simulink model "extra2 - Copy"  (R2017a)
settings: Solver=VariableStepAuto  StartTime=0.0  StopTime=10.0  RelTol=1e-3
libraries: hdlsllib x20, simulink x10
settings Model: Creator=wachala.j  LastModifiedBy=wachala.j
settings OptimizationCC: BlockReduction=off  ConditionallyExecuteInputs=off  DefaultParameterBehavior=Inlined
settings DebuggingCC: AlgebraicLoopMsg=error
settings HardwareCC: ProdBitPerPointer=32  ProdBitPerSizeT=32  ProdBitPerPtrDiffT=32  ProdLargestAtomicFloat=None  ProdIntDivRoundTo=Undefined  ProdEndianess=Unspecified  ProdWordSize=32  ProdHWDeviceType=ASIC/FPGA->ASIC/FPGA  ProdEqTarget=off

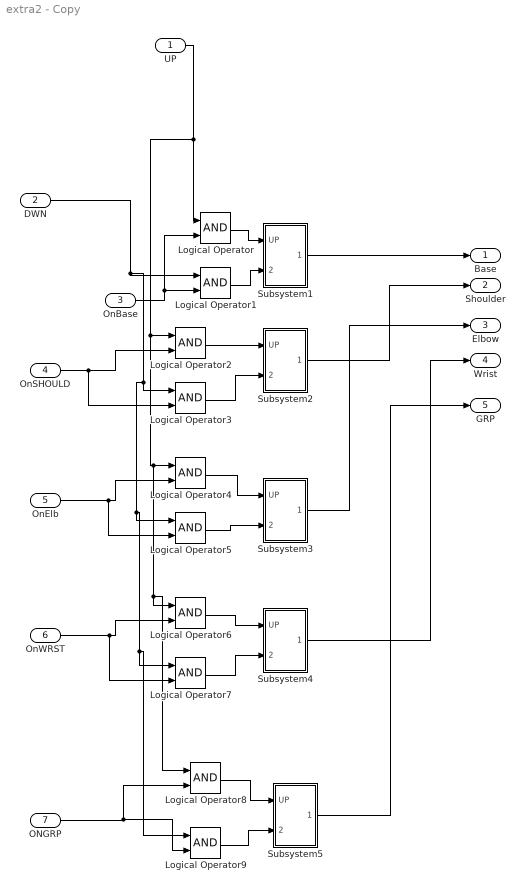
== system extra2 - Copy ==
  UP : Inport
  DWN : Inport  Port=2
  OnBase : Inport  Port=3
  OnSHOULD : Inport  Port=4
  OnElb : Inport  Port=5
  OnWRST : Inport  Port=6
  ONGRP : Inport  Port=7
  Logical Operator{,1..9} (10 alike) : Logic  AllPortsSameDT=off  OutDataTypeStr=boolean
  Subsystem1 : Subsystem
  Subsystem2 : Subsystem
  Subsystem3 : Subsystem
  Subsystem4 : Subsystem
  Subsystem5 : Subsystem
  Base : Outport  OutDataTypeStr=boolean
  "Shoulder " : Outport  Port=2  OutDataTypeStr=boolean
  Elbow : Outport  Port=3  OutDataTypeStr=boolean
  Wrist : Outport  Port=4  OutDataTypeStr=boolean
  GRP : Outport  Port=5  OutDataTypeStr=boolean
  wires:
  UP/1 -> Logical Operator8/1, Logical Operator6/1, Logical Operator4/1, Logical Operator2/1, Logical Operator/1
  OnBase/1 -> Logical Operator1/2, Logical Operator/2
  DWN/1 -> Logical Operator9/1, Logical Operator7/1, Logical Operator5/1, Logical Operator3/1, Logical Operator1/1
  Logical Operator1/1 -> Subsystem1/2(DWN)
  Logical Operator/1 -> Subsystem1/1(UP)
  Subsystem1/1(PWM) -> Base/1
  ONGRP/1 -> Logical Operator9/2, Logical Operator8/2
  OnWRST/1 -> Logical Operator7/2, Logical Operator6/2
  OnElb/1 -> Logical Operator5/2, Logical Operator4/2
  OnSHOULD/1 -> Logical Operator3/2, Logical Operator2/2
  Logical Operator8/1 -> Subsystem5/1(UP)
  Logical Operator9/1 -> Subsystem5/2(DWN)
  Logical Operator7/1 -> Subsystem4/2(DWN)
  Logical Operator6/1 -> Subsystem4/1(UP)
  Logical Operator5/1 -> Subsystem3/2(DWN)
  Logical Operator4/1 -> Subsystem3/1(UP)
  Logical Operator3/1 -> Subsystem2/2(DWN)
  Logical Operator2/1 -> Subsystem2/1(UP)
  Subsystem2/1(PWM) -> "Shoulder "/1
  Subsystem3/1(PWM) -> Elbow/1
  Subsystem4/1(PWM) -> Wrist/1
  Subsystem5/1(PWM) -> GRP/1

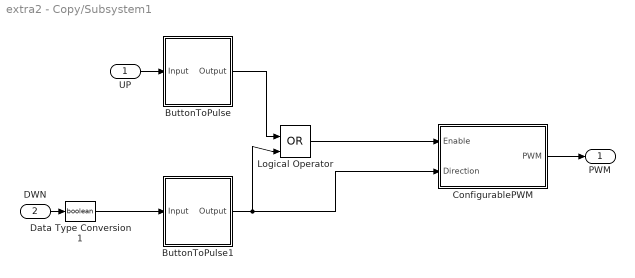
== system extra2 - Copy/Subsystem1 ==
  UP : Inport
  DWN : Inport  Port=2
  ButtonToPulse : Subsystem
  ButtonToPulse1 : Subsystem
  ConfigurablePWM : Subsystem
  Data Type Conversion1 : DataTypeConversion  OutDataTypeStr=boolean
  Logical Operator : Logic  Operator=OR  IconShape=distinctive  AllPortsSameDT=off  OutDataTypeStr=boolean
  PWM : Outport  OutDataTypeStr=boolean
  wires:
  ButtonToPulse1/1(Output) -> Logical Operator/2, ConfigurablePWM/2(Direction)
  Data Type Conversion1/1 -> ButtonToPulse1/1(Input)
  ButtonToPulse/1(Output) -> Logical Operator/1
  UP/1 -> ButtonToPulse/1(Input)
  DWN/1 -> Data Type Conversion1/1
  Logical Operator/1 -> ConfigurablePWM/1(Enable)
  ConfigurablePWM/1(PWM) -> PWM/1

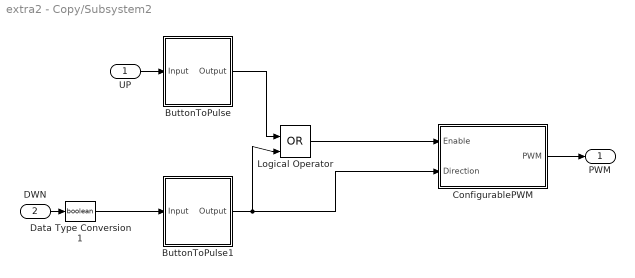
== system extra2 - Copy/Subsystem2 ==
  UP : Inport
  DWN : Inport  Port=2
  ButtonToPulse : Subsystem
  ButtonToPulse1 : Subsystem
  ConfigurablePWM : Subsystem
  Data Type Conversion1 : DataTypeConversion  OutDataTypeStr=boolean
  Logical Operator : Logic  Operator=OR  IconShape=distinctive  AllPortsSameDT=off  OutDataTypeStr=boolean
  PWM : Outport  OutDataTypeStr=boolean
  wires:
  ButtonToPulse1/1(Output) -> Logical Operator/2, ConfigurablePWM/2(Direction)
  Data Type Conversion1/1 -> ButtonToPulse1/1(Input)
  ButtonToPulse/1(Output) -> Logical Operator/1
  UP/1 -> ButtonToPulse/1(Input)
  DWN/1 -> Data Type Conversion1/1
  Logical Operator/1 -> ConfigurablePWM/1(Enable)
  ConfigurablePWM/1(PWM) -> PWM/1

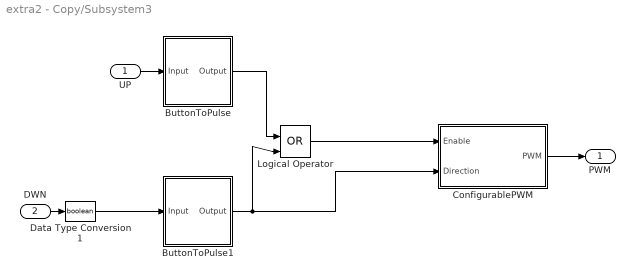
== system extra2 - Copy/Subsystem3 ==
  UP : Inport
  DWN : Inport  Port=2
  ButtonToPulse : Subsystem
  ButtonToPulse1 : Subsystem
  ConfigurablePWM : Subsystem
  Data Type Conversion1 : DataTypeConversion  OutDataTypeStr=boolean
  Logical Operator : Logic  Operator=OR  IconShape=distinctive  AllPortsSameDT=off  OutDataTypeStr=boolean
  PWM : Outport  OutDataTypeStr=boolean
  wires:
  ButtonToPulse1/1(Output) -> Logical Operator/2, ConfigurablePWM/2(Direction)
  Data Type Conversion1/1 -> ButtonToPulse1/1(Input)
  ButtonToPulse/1(Output) -> Logical Operator/1
  UP/1 -> ButtonToPulse/1(Input)
  DWN/1 -> Data Type Conversion1/1
  Logical Operator/1 -> ConfigurablePWM/1(Enable)
  ConfigurablePWM/1(PWM) -> PWM/1

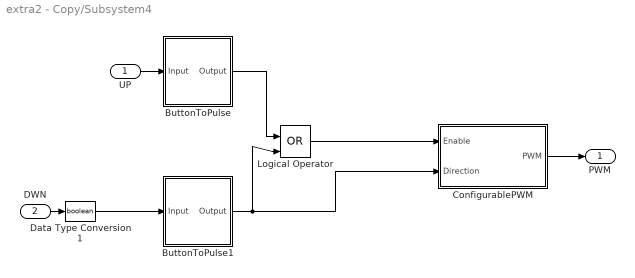
== system extra2 - Copy/Subsystem4 ==
  UP : Inport
  DWN : Inport  Port=2
  ButtonToPulse : Subsystem
  ButtonToPulse1 : Subsystem
  ConfigurablePWM : Subsystem
  Data Type Conversion1 : DataTypeConversion  OutDataTypeStr=boolean
  Logical Operator : Logic  Operator=OR  IconShape=distinctive  AllPortsSameDT=off  OutDataTypeStr=boolean
  PWM : Outport  OutDataTypeStr=boolean
  wires:
  ButtonToPulse1/1(Output) -> Logical Operator/2, ConfigurablePWM/2(Direction)
  Data Type Conversion1/1 -> ButtonToPulse1/1(Input)
  ButtonToPulse/1(Output) -> Logical Operator/1
  UP/1 -> ButtonToPulse/1(Input)
  DWN/1 -> Data Type Conversion1/1
  Logical Operator/1 -> ConfigurablePWM/1(Enable)
  ConfigurablePWM/1(PWM) -> PWM/1

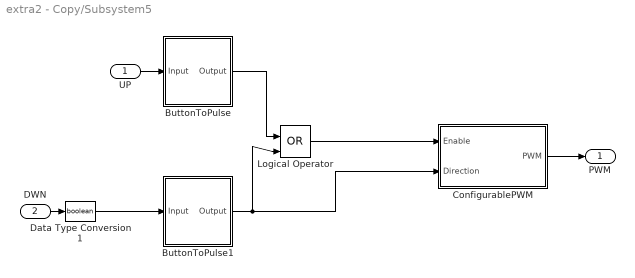
== system extra2 - Copy/Subsystem5 ==
  UP : Inport
  DWN : Inport  Port=2
  ButtonToPulse : Subsystem
  ButtonToPulse1 : Subsystem
  ConfigurablePWM : Subsystem
  Data Type Conversion1 : DataTypeConversion  OutDataTypeStr=boolean
  Logical Operator : Logic  Operator=OR  IconShape=distinctive  AllPortsSameDT=off  OutDataTypeStr=boolean
  PWM : Outport  OutDataTypeStr=boolean
  wires:
  ButtonToPulse1/1(Output) -> Logical Operator/2, ConfigurablePWM/2(Direction)
  Data Type Conversion1/1 -> ButtonToPulse1/1(Input)
  ButtonToPulse/1(Output) -> Logical Operator/1
  UP/1 -> ButtonToPulse/1(Input)
  DWN/1 -> Data Type Conversion1/1
  Logical Operator/1 -> ConfigurablePWM/1(Enable)
  ConfigurablePWM/1(PWM) -> PWM/1

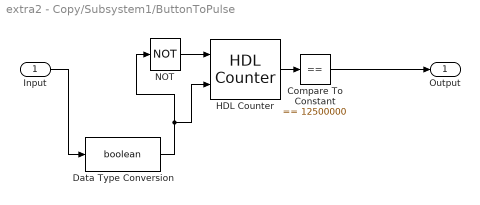
== system extra2 - Copy/Subsystem1/ButtonToPulse ==
  Input : Inport
  Compare To Constant : simulink/Logic and Bit Operations/Compare To Constant  relop===  const=12500000  OutDataTypeStr=boolean
  Data Type Conversion : DataTypeConversion  OutDataTypeStr=boolean
  HDL Counter : hdlsllib/HDL Operations/HDL Counter  CountType=Count limited  CountInit=0  CountStep=1  CountMax=50000000  CountFromType=Initial value  CountFrom=0  CountResetPort=on  CountLoadPort=off  CountEnbPort=on  CountDirPort=off  CountDataType=Unsigned  CountWordLen=32  CountFracLen=0  CountSampTime=1
      settings: SourceProductName=HDL Coder  SourceProductBaseCode=HD
  NOT : Logic  Operator=NOT  IconShape=distinctive  AllPortsSameDT=off  OutDataTypeStr=boolean
  Output : Outport
  wires:
  NOT/1 -> HDL Counter/1
  Data Type Conversion/1 -> HDL Counter/2, NOT/1
  HDL Counter/1 -> Compare To Constant/1
  Input/1 -> Data Type Conversion/1
  Compare To Constant/1 -> Output/1

== system extra2 - Copy/Subsystem1/ButtonToPulse1 ==
  Input : Inport
  Compare To Constant : simulink/Logic and Bit Operations/Compare To Constant  relop===  const=12500000  OutDataTypeStr=boolean
  Data Type Conversion : DataTypeConversion  OutDataTypeStr=boolean
  HDL Counter : hdlsllib/HDL Operations/HDL Counter  CountType=Count limited  CountInit=0  CountStep=1  CountMax=50000000  CountFromType=Initial value  CountFrom=0  CountResetPort=on  CountLoadPort=off  CountEnbPort=on  CountDirPort=off  CountDataType=Unsigned  CountWordLen=32  CountFracLen=0  CountSampTime=1
      settings: SourceProductName=HDL Coder  SourceProductBaseCode=HD
  NOT : Logic  Operator=NOT  IconShape=distinctive  AllPortsSameDT=off  OutDataTypeStr=boolean
  Output : Outport
  wires:
  NOT/1 -> HDL Counter/1
  Data Type Conversion/1 -> HDL Counter/2, NOT/1
  HDL Counter/1 -> Compare To Constant/1
  Input/1 -> Data Type Conversion/1
  Compare To Constant/1 -> Output/1

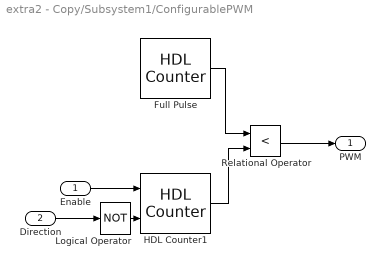
== system extra2 - Copy/Subsystem1/ConfigurablePWM ==
  Enable : Inport  OutDataTypeStr=boolean
  Direction : Inport  Port=2  OutDataTypeStr=boolean
  Full Pulse : hdlsllib/HDL Operations/HDL Counter  CountType=Count limited  CountInit=0  CountStep=1  CountMax=1000000  CountFromType=Initial value  CountFrom=0  CountResetPort=off  CountLoadPort=off  CountEnbPort=off  CountDirPort=off  CountDataType=Unsigned  CountWordLen=32  CountFracLen=0  CountSampTime=1
      settings: SourceProductName=HDL Coder  SourceProductBaseCode=HD
  HDL Counter1 : hdlsllib/HDL Operations/HDL Counter  CountType=Count limited  CountInit=30000  CountStep=6000  CountMax=120000  CountFromType=Initial value  CountFrom=30000  CountResetPort=off  CountLoadPort=off  CountEnbPort=on  CountDirPort=on  CountDataType=Unsigned  CountWordLen=32  CountFracLen=0  CountSampTime=1
      settings: SourceProductName=HDL Coder  SourceProductBaseCode=HD
  Logical Operator : Logic  Operator=NOT  IconShape=distinctive  AllPortsSameDT=off  OutDataTypeStr=boolean
  Relational Operator : RelationalOperator  Operator=<  OutDataTypeStr=boolean  RndMeth=Simplest
  PWM : Outport
  wires:
  Relational Operator/1 -> PWM/1
  HDL Counter1/1 -> Relational Operator/2
  Full Pulse/1 -> Relational Operator/1
  Enable/1 -> HDL Counter1/1
  Direction/1 -> Logical Operator/1
  Logical Operator/1 -> HDL Counter1/2

== system extra2 - Copy/Subsystem2/ButtonToPulse ==
  Input : Inport
  Compare To Constant : simulink/Logic and Bit Operations/Compare To Constant  relop===  const=12500000  OutDataTypeStr=boolean
  Data Type Conversion : DataTypeConversion  OutDataTypeStr=boolean
  HDL Counter : hdlsllib/HDL Operations/HDL Counter  CountType=Count limited  CountInit=0  CountStep=1  CountMax=50000000  CountFromType=Initial value  CountFrom=0  CountResetPort=on  CountLoadPort=off  CountEnbPort=on  CountDirPort=off  CountDataType=Unsigned  CountWordLen=32  CountFracLen=0  CountSampTime=1
      settings: SourceProductName=HDL Coder  SourceProductBaseCode=HD
  NOT : Logic  Operator=NOT  IconShape=distinctive  AllPortsSameDT=off  OutDataTypeStr=boolean
  Output : Outport
  wires:
  NOT/1 -> HDL Counter/1
  Data Type Conversion/1 -> HDL Counter/2, NOT/1
  HDL Counter/1 -> Compare To Constant/1
  Input/1 -> Data Type Conversion/1
  Compare To Constant/1 -> Output/1

== system extra2 - Copy/Subsystem2/ButtonToPulse1 ==
  Input : Inport
  Compare To Constant : simulink/Logic and Bit Operations/Compare To Constant  relop===  const=12500000  OutDataTypeStr=boolean
  Data Type Conversion : DataTypeConversion  OutDataTypeStr=boolean
  HDL Counter : hdlsllib/HDL Operations/HDL Counter  CountType=Count limited  CountInit=0  CountStep=1  CountMax=50000000  CountFromType=Initial value  CountFrom=0  CountResetPort=on  CountLoadPort=off  CountEnbPort=on  CountDirPort=off  CountDataType=Unsigned  CountWordLen=32  CountFracLen=0  CountSampTime=1
      settings: SourceProductName=HDL Coder  SourceProductBaseCode=HD
  NOT : Logic  Operator=NOT  IconShape=distinctive  AllPortsSameDT=off  OutDataTypeStr=boolean
  Output : Outport
  wires:
  NOT/1 -> HDL Counter/1
  Data Type Conversion/1 -> HDL Counter/2, NOT/1
  HDL Counter/1 -> Compare To Constant/1
  Input/1 -> Data Type Conversion/1
  Compare To Constant/1 -> Output/1

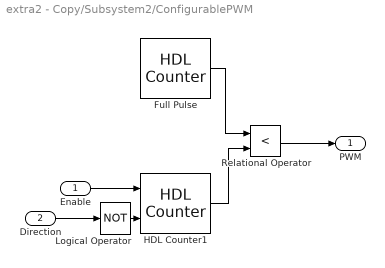
== system extra2 - Copy/Subsystem2/ConfigurablePWM ==
  Enable : Inport  OutDataTypeStr=boolean
  Direction : Inport  Port=2  OutDataTypeStr=boolean
  Full Pulse : hdlsllib/HDL Operations/HDL Counter  CountType=Count limited  CountInit=0  CountStep=1  CountMax=1000000  CountFromType=Initial value  CountFrom=0  CountResetPort=off  CountLoadPort=off  CountEnbPort=off  CountDirPort=off  CountDataType=Unsigned  CountWordLen=32  CountFracLen=0  CountSampTime=1
      settings: SourceProductName=HDL Coder  SourceProductBaseCode=HD
  HDL Counter1 : hdlsllib/HDL Operations/HDL Counter  CountType=Count limited  CountInit=30000  CountStep=6000  CountMax=120000  CountFromType=Initial value  CountFrom=30000  CountResetPort=off  CountLoadPort=off  CountEnbPort=on  CountDirPort=on  CountDataType=Unsigned  CountWordLen=32  CountFracLen=0  CountSampTime=1
      settings: SourceProductName=HDL Coder  SourceProductBaseCode=HD
  Logical Operator : Logic  Operator=NOT  IconShape=distinctive  AllPortsSameDT=off  OutDataTypeStr=boolean
  Relational Operator : RelationalOperator  Operator=<  OutDataTypeStr=boolean  RndMeth=Simplest
  PWM : Outport
  wires:
  Relational Operator/1 -> PWM/1
  HDL Counter1/1 -> Relational Operator/2
  Full Pulse/1 -> Relational Operator/1
  Enable/1 -> HDL Counter1/1
  Direction/1 -> Logical Operator/1
  Logical Operator/1 -> HDL Counter1/2

== system extra2 - Copy/Subsystem3/ButtonToPulse ==
  Input : Inport
  Compare To Constant : simulink/Logic and Bit Operations/Compare To Constant  relop===  const=12500000  OutDataTypeStr=boolean
  Data Type Conversion : DataTypeConversion  OutDataTypeStr=boolean
  HDL Counter : hdlsllib/HDL Operations/HDL Counter  CountType=Count limited  CountInit=0  CountStep=1  CountMax=50000000  CountFromType=Initial value  CountFrom=0  CountResetPort=on  CountLoadPort=off  CountEnbPort=on  CountDirPort=off  CountDataType=Unsigned  CountWordLen=32  CountFracLen=0  CountSampTime=1
      settings: SourceProductName=HDL Coder  SourceProductBaseCode=HD
  NOT : Logic  Operator=NOT  IconShape=distinctive  AllPortsSameDT=off  OutDataTypeStr=boolean
  Output : Outport
  wires:
  NOT/1 -> HDL Counter/1
  Data Type Conversion/1 -> HDL Counter/2, NOT/1
  HDL Counter/1 -> Compare To Constant/1
  Input/1 -> Data Type Conversion/1
  Compare To Constant/1 -> Output/1

== system extra2 - Copy/Subsystem3/ButtonToPulse1 ==
  Input : Inport
  Compare To Constant : simulink/Logic and Bit Operations/Compare To Constant  relop===  const=12500000  OutDataTypeStr=boolean
  Data Type Conversion : DataTypeConversion  OutDataTypeStr=boolean
  HDL Counter : hdlsllib/HDL Operations/HDL Counter  CountType=Count limited  CountInit=0  CountStep=1  CountMax=50000000  CountFromType=Initial value  CountFrom=0  CountResetPort=on  CountLoadPort=off  CountEnbPort=on  CountDirPort=off  CountDataType=Unsigned  CountWordLen=32  CountFracLen=0  CountSampTime=1
      settings: SourceProductName=HDL Coder  SourceProductBaseCode=HD
  NOT : Logic  Operator=NOT  IconShape=distinctive  AllPortsSameDT=off  OutDataTypeStr=boolean
  Output : Outport
  wires:
  NOT/1 -> HDL Counter/1
  Data Type Conversion/1 -> HDL Counter/2, NOT/1
  HDL Counter/1 -> Compare To Constant/1
  Input/1 -> Data Type Conversion/1
  Compare To Constant/1 -> Output/1

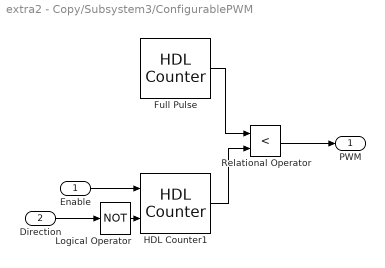
== system extra2 - Copy/Subsystem3/ConfigurablePWM ==
  Enable : Inport  OutDataTypeStr=boolean
  Direction : Inport  Port=2  OutDataTypeStr=boolean
  Full Pulse : hdlsllib/HDL Operations/HDL Counter  CountType=Count limited  CountInit=0  CountStep=1  CountMax=1000000  CountFromType=Initial value  CountFrom=0  CountResetPort=off  CountLoadPort=off  CountEnbPort=off  CountDirPort=off  CountDataType=Unsigned  CountWordLen=32  CountFracLen=0  CountSampTime=1
      settings: SourceProductName=HDL Coder  SourceProductBaseCode=HD
  HDL Counter1 : hdlsllib/HDL Operations/HDL Counter  CountType=Count limited  CountInit=30000  CountStep=6000  CountMax=120000  CountFromType=Initial value  CountFrom=30000  CountResetPort=off  CountLoadPort=off  CountEnbPort=on  CountDirPort=on  CountDataType=Unsigned  CountWordLen=32  CountFracLen=0  CountSampTime=1
      settings: SourceProductName=HDL Coder  SourceProductBaseCode=HD
  Logical Operator : Logic  Operator=NOT  IconShape=distinctive  AllPortsSameDT=off  OutDataTypeStr=boolean
  Relational Operator : RelationalOperator  Operator=<  OutDataTypeStr=boolean  RndMeth=Simplest
  PWM : Outport
  wires:
  Relational Operator/1 -> PWM/1
  HDL Counter1/1 -> Relational Operator/2
  Full Pulse/1 -> Relational Operator/1
  Enable/1 -> HDL Counter1/1
  Direction/1 -> Logical Operator/1
  Logical Operator/1 -> HDL Counter1/2

== system extra2 - Copy/Subsystem4/ButtonToPulse ==
  Input : Inport
  Compare To Constant : simulink/Logic and Bit Operations/Compare To Constant  relop===  const=12500000  OutDataTypeStr=boolean
  Data Type Conversion : DataTypeConversion  OutDataTypeStr=boolean
  HDL Counter : hdlsllib/HDL Operations/HDL Counter  CountType=Count limited  CountInit=0  CountStep=1  CountMax=50000000  CountFromType=Initial value  CountFrom=0  CountResetPort=on  CountLoadPort=off  CountEnbPort=on  CountDirPort=off  CountDataType=Unsigned  CountWordLen=32  CountFracLen=0  CountSampTime=1
      settings: SourceProductName=HDL Coder  SourceProductBaseCode=HD
  NOT : Logic  Operator=NOT  IconShape=distinctive  AllPortsSameDT=off  OutDataTypeStr=boolean
  Output : Outport
  wires:
  NOT/1 -> HDL Counter/1
  Data Type Conversion/1 -> HDL Counter/2, NOT/1
  HDL Counter/1 -> Compare To Constant/1
  Input/1 -> Data Type Conversion/1
  Compare To Constant/1 -> Output/1

== system extra2 - Copy/Subsystem4/ButtonToPulse1 ==
  Input : Inport
  Compare To Constant : simulink/Logic and Bit Operations/Compare To Constant  relop===  const=12500000  OutDataTypeStr=boolean
  Data Type Conversion : DataTypeConversion  OutDataTypeStr=boolean
  HDL Counter : hdlsllib/HDL Operations/HDL Counter  CountType=Count limited  CountInit=0  CountStep=1  CountMax=50000000  CountFromType=Initial value  CountFrom=0  CountResetPort=on  CountLoadPort=off  CountEnbPort=on  CountDirPort=off  CountDataType=Unsigned  CountWordLen=32  CountFracLen=0  CountSampTime=1
      settings: SourceProductName=HDL Coder  SourceProductBaseCode=HD
  NOT : Logic  Operator=NOT  IconShape=distinctive  AllPortsSameDT=off  OutDataTypeStr=boolean
  Output : Outport
  wires:
  NOT/1 -> HDL Counter/1
  Data Type Conversion/1 -> HDL Counter/2, NOT/1
  HDL Counter/1 -> Compare To Constant/1
  Input/1 -> Data Type Conversion/1
  Compare To Constant/1 -> Output/1

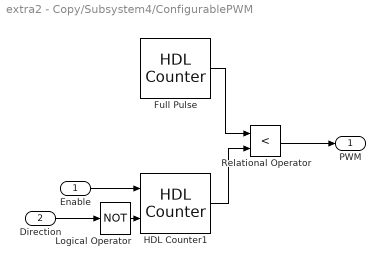
== system extra2 - Copy/Subsystem4/ConfigurablePWM ==
  Enable : Inport  OutDataTypeStr=boolean
  Direction : Inport  Port=2  OutDataTypeStr=boolean
  Full Pulse : hdlsllib/HDL Operations/HDL Counter  CountType=Count limited  CountInit=0  CountStep=1  CountMax=1000000  CountFromType=Initial value  CountFrom=0  CountResetPort=off  CountLoadPort=off  CountEnbPort=off  CountDirPort=off  CountDataType=Unsigned  CountWordLen=32  CountFracLen=0  CountSampTime=1
      settings: SourceProductName=HDL Coder  SourceProductBaseCode=HD
  HDL Counter1 : hdlsllib/HDL Operations/HDL Counter  CountType=Count limited  CountInit=30000  CountStep=6000  CountMax=120000  CountFromType=Initial value  CountFrom=30000  CountResetPort=off  CountLoadPort=off  CountEnbPort=on  CountDirPort=on  CountDataType=Unsigned  CountWordLen=32  CountFracLen=0  CountSampTime=1
      settings: SourceProductName=HDL Coder  SourceProductBaseCode=HD
  Logical Operator : Logic  Operator=NOT  IconShape=distinctive  AllPortsSameDT=off  OutDataTypeStr=boolean
  Relational Operator : RelationalOperator  Operator=<  OutDataTypeStr=boolean  RndMeth=Simplest
  PWM : Outport
  wires:
  Relational Operator/1 -> PWM/1
  HDL Counter1/1 -> Relational Operator/2
  Full Pulse/1 -> Relational Operator/1
  Enable/1 -> HDL Counter1/1
  Direction/1 -> Logical Operator/1
  Logical Operator/1 -> HDL Counter1/2

== system extra2 - Copy/Subsystem5/ButtonToPulse ==
  Input : Inport
  Compare To Constant : simulink/Logic and Bit Operations/Compare To Constant  relop===  const=12500000  OutDataTypeStr=boolean
  Data Type Conversion : DataTypeConversion  OutDataTypeStr=boolean
  HDL Counter : hdlsllib/HDL Operations/HDL Counter  CountType=Count limited  CountInit=0  CountStep=1  CountMax=50000000  CountFromType=Initial value  CountFrom=0  CountResetPort=on  CountLoadPort=off  CountEnbPort=on  CountDirPort=off  CountDataType=Unsigned  CountWordLen=32  CountFracLen=0  CountSampTime=1
      settings: SourceProductName=HDL Coder  SourceProductBaseCode=HD
  NOT : Logic  Operator=NOT  IconShape=distinctive  AllPortsSameDT=off  OutDataTypeStr=boolean
  Output : Outport
  wires:
  NOT/1 -> HDL Counter/1
  Data Type Conversion/1 -> HDL Counter/2, NOT/1
  HDL Counter/1 -> Compare To Constant/1
  Input/1 -> Data Type Conversion/1
  Compare To Constant/1 -> Output/1

== system extra2 - Copy/Subsystem5/ButtonToPulse1 ==
  Input : Inport
  Compare To Constant : simulink/Logic and Bit Operations/Compare To Constant  relop===  const=12500000  OutDataTypeStr=boolean
  Data Type Conversion : DataTypeConversion  OutDataTypeStr=boolean
  HDL Counter : hdlsllib/HDL Operations/HDL Counter  CountType=Count limited  CountInit=0  CountStep=1  CountMax=50000000  CountFromType=Initial value  CountFrom=0  CountResetPort=on  CountLoadPort=off  CountEnbPort=on  CountDirPort=off  CountDataType=Unsigned  CountWordLen=32  CountFracLen=0  CountSampTime=1
      settings: SourceProductName=HDL Coder  SourceProductBaseCode=HD
  NOT : Logic  Operator=NOT  IconShape=distinctive  AllPortsSameDT=off  OutDataTypeStr=boolean
  Output : Outport
  wires:
  NOT/1 -> HDL Counter/1
  Data Type Conversion/1 -> HDL Counter/2, NOT/1
  HDL Counter/1 -> Compare To Constant/1
  Input/1 -> Data Type Conversion/1
  Compare To Constant/1 -> Output/1

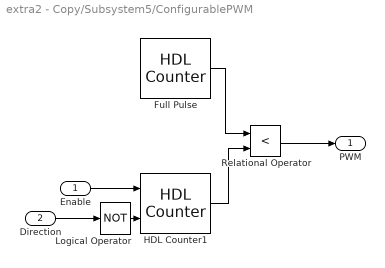
== system extra2 - Copy/Subsystem5/ConfigurablePWM ==
  Enable : Inport  OutDataTypeStr=boolean
  Direction : Inport  Port=2  OutDataTypeStr=boolean
  Full Pulse : hdlsllib/HDL Operations/HDL Counter  CountType=Count limited  CountInit=0  CountStep=1  CountMax=1000000  CountFromType=Initial value  CountFrom=0  CountResetPort=off  CountLoadPort=off  CountEnbPort=off  CountDirPort=off  CountDataType=Unsigned  CountWordLen=32  CountFracLen=0  CountSampTime=1
      settings: SourceProductName=HDL Coder  SourceProductBaseCode=HD
  HDL Counter1 : hdlsllib/HDL Operations/HDL Counter  CountType=Count limited  CountInit=30000  CountStep=6000  CountMax=120000  CountFromType=Initial value  CountFrom=30000  CountResetPort=off  CountLoadPort=off  CountEnbPort=on  CountDirPort=on  CountDataType=Unsigned  CountWordLen=32  CountFracLen=0  CountSampTime=1
      settings: SourceProductName=HDL Coder  SourceProductBaseCode=HD
  Logical Operator : Logic  Operator=NOT  IconShape=distinctive  AllPortsSameDT=off  OutDataTypeStr=boolean
  Relational Operator : RelationalOperator  Operator=<  OutDataTypeStr=boolean  RndMeth=Simplest
  PWM : Outport
  wires:
  Relational Operator/1 -> PWM/1
  HDL Counter1/1 -> Relational Operator/2
  Full Pulse/1 -> Relational Operator/1
  Enable/1 -> HDL Counter1/1
  Direction/1 -> Logical Operator/1
  Logical Operator/1 -> HDL Counter1/2
